simulink model "two"  (R2014a)
settings: Solver=ode45  StartTime=0.0  StopTime=25  MaxStep=0.001  MinStep=0.0001  RelTol=1e-3
settings Model: Creator=trigg  LastModifiedBy=trigg

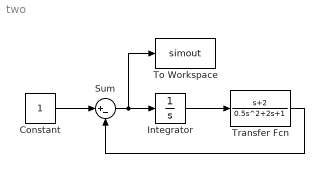
== system two ==
  Constant : Constant
  Integrator : Integrator  InitialCondition=10
  Sum : Sum  Inputs=|+-
  To Workspace : ToWorkspace  VariableName=simout  SaveFormat=Timeseries  SampleTime=-1
  Transfer Fcn : TransferFcn  Numerator=[1 2]  Denominator=[0.5 2 1]
  wires:
  Constant/1 -> Sum/1
  Sum/1 -> To Workspace/1, Integrator/1
  Integrator/1 -> Transfer Fcn/1
  Transfer Fcn/1 -> Sum/2
